simulink model "W01_Base_Map_cs"  (R2019a)
settings: Solver=FixedStepDiscrete  StartTime=0.0  StopTime=inf  FixedStep=1/20  RelTol=1e-3
PreLoadFcn:
  | mbxruntime.callbacks.PreLoadFcn(bdroot);
  | check_NUTS_defined
  | model_closed = 0;
  | assignin('base',['model_closed_' bdroot],false);
PostLoadFcn:
  | mbxruntime.callbacks.PostLoadFcn(bdroot);
InitFcn:
  | mbxruntime.callbacks.InitFcn(bdroot);
StartFcn:
  | mbxruntime.callbacks.StartFcn(bdroot);
StopFcn:
  | mbxruntime.callbacks.StopFcn(bdroot);;
  | 
model workspace: external: MAT-File .\W01_Base_Map_cs_hws.mat (data not in the file)
undefined symbols (not defined in the file or in its folder): DiscIntNeverNeededParam, Header, mbxruntime, Orientation, Poses, Poses_SL_Info, Position, tabledata, W01_Base_Map_cs_328ec7e3a8cd5b54, W01_Base_Map_cs_514c2dea2cdbe680, W01_Base_Map_cs_51d6e6e467bedba1, W01_Base_Map_cs_563ebd29d1fd6c09, W01_Base_Map_cs_57ea59d0358dab77, W01_Base_Map_cs_9538d35a279fbe4e, W01_Base_Map_cs_9f504bb84aebc2fd, W01_Base_Map_cs_a242ed7539861165, W01_Base_Map_cs_Audi_A8_Sedan_1_Path_pathUniqueID, W01_Base_Map_cs_b5931a786e299506, W01_Base_Map_cs_b7f45a070fa6e639, W01_Base_Map_cs_c02beb48492dde12, W01_Base_Map_cs_cf83ac8e8b053cbf, W01_Base_Map_cs_Child_RegularAni_1_Path_pathUniqueID, W01_Base_Map_cs_Child_RegularAni_2_Path_pathUniqueID, W01_Base_Map_cs_Citroen_C3_Hatchback_1_Path_pathUniqueID, W01_Base_Map_cs_d4423fcf1c0d6fc4, W01_Base_Map_cs_Female_RegularAni_1_Path_pathUniqueID, W01_Base_Map_cs_Male_RegularAni_1_Path_pathUniqueID, W01_Base_Map_cs_Male_RegularAni_2_Path_pathUniqueID
libraries: simulink_extras x30, adeye_lib x16, simulink x10, robotlib x4, sharedtransform x2, PreScanSimulinkLibrary x2, PreScanUsefulBlocks x1
(part 7 of 8)

== system W01_Base_Map_cs/TrafficLightRoadSideNL_1/Green_Mux ==
  MSCD [Cd] : Inport
  Position (xyz) [m] : Inport  Port=2
  Orientation (RPY) [deg] : Inport  Port=3
  Color [-] : Inport  Port=4
  TextureResourceID [-] : Inport  Port=5
  Bus Creator : BusCreator  Inputs='Intensity','Position','Orientation','Color','TextureResourceID'  OutDataTypeStr=Bus: PRESCAN_VISULIGHTACTUATOR_DATA  NonVirtualBus=on
  Bus Creator1 : BusCreator  Inputs=3  OutDataTypeStr=Bus: PRESCAN_RGB_DATA  NonVirtualBus=on
  Bus Creator2 : BusCreator  Inputs=3  OutDataTypeStr=Bus: PRESCAN_RPY_DATA  NonVirtualBus=on
  Bus Creator3 : BusCreator  Inputs=3  OutDataTypeStr=Bus: PRESCAN_XYZ_DATA  NonVirtualBus=on
  Data Type Conversion : DataTypeConversion  OutDataTypeStr=int32  RndMeth=Nearest
  Degrees to Radians : simulink_extras/Transformations/Degrees to Radians
  Demux : Demux  Outputs=3
  Demux1 : Demux  Outputs=3
  Demux2 : Demux  Outputs=3
  Lights : Outport
  wires:
  TextureResourceID [-]/1 -> Data Type Conversion/1  "TextureResourceID"
  MSCD [Cd]/1 -> Bus Creator/1  "Intensity"
  Bus Creator/1 -> Lights/1
  Demux/1 -> Bus Creator1/1  "R"
  Demux/2 -> Bus Creator1/2  "G"
  Demux/3 -> Bus Creator1/3  "B"
  Color [-]/1 -> Demux/1  "Color"
  Bus Creator1/1 -> Bus Creator/4  "Color"
  Demux1/1 -> Bus Creator2/1  "Roll"
  Demux1/2 -> Bus Creator2/2  "Pitch"
  Demux1/3 -> Bus Creator2/3  "Yaw"
  Orientation (RPY) [deg]/1 -> Degrees to Radians/1  "Orientation"
  Bus Creator2/1 -> Bus Creator/3  "Orientation"
  Demux2/1 -> Bus Creator3/1  "X"
  Demux2/2 -> Bus Creator3/2  "Y"
  Demux2/3 -> Bus Creator3/3  "Z"
  Position (xyz) [m]/1 -> Demux2/1  "Position"
  Bus Creator3/1 -> Bus Creator/2  "Position"
  Data Type Conversion/1 -> Bus Creator/5  "TextureResourceID"
  Degrees to Radians/1 -> Demux1/1

== system W01_Base_Map_cs/TrafficLightRoadSideNL_1/Orange_Mux ==
  MSCD [Cd] : Inport
  Position (xyz) [m] : Inport  Port=2
  Orientation (RPY) [deg] : Inport  Port=3
  Color [-] : Inport  Port=4
  TextureResourceID [-] : Inport  Port=5
  Bus Creator : BusCreator  Inputs='Intensity','Position','Orientation','Color','TextureResourceID'  OutDataTypeStr=Bus: PRESCAN_VISULIGHTACTUATOR_DATA  NonVirtualBus=on
  Bus Creator1 : BusCreator  Inputs=3  OutDataTypeStr=Bus: PRESCAN_RGB_DATA  NonVirtualBus=on
  Bus Creator2 : BusCreator  Inputs=3  OutDataTypeStr=Bus: PRESCAN_RPY_DATA  NonVirtualBus=on
  Bus Creator3 : BusCreator  Inputs=3  OutDataTypeStr=Bus: PRESCAN_XYZ_DATA  NonVirtualBus=on
  Data Type Conversion : DataTypeConversion  OutDataTypeStr=int32  RndMeth=Nearest
  Degrees to Radians : simulink_extras/Transformations/Degrees to Radians
  Demux : Demux  Outputs=3
  Demux1 : Demux  Outputs=3
  Demux2 : Demux  Outputs=3
  Lights : Outport
  wires:
  TextureResourceID [-]/1 -> Data Type Conversion/1  "TextureResourceID"
  MSCD [Cd]/1 -> Bus Creator/1  "Intensity"
  Bus Creator/1 -> Lights/1
  Demux/1 -> Bus Creator1/1  "R"
  Demux/2 -> Bus Creator1/2  "G"
  Demux/3 -> Bus Creator1/3  "B"
  Color [-]/1 -> Demux/1  "Color"
  Bus Creator1/1 -> Bus Creator/4  "Color"
  Demux1/1 -> Bus Creator2/1  "Roll"
  Demux1/2 -> Bus Creator2/2  "Pitch"
  Demux1/3 -> Bus Creator2/3  "Yaw"
  Orientation (RPY) [deg]/1 -> Degrees to Radians/1  "Orientation"
  Bus Creator2/1 -> Bus Creator/3  "Orientation"
  Demux2/1 -> Bus Creator3/1  "X"
  Demux2/2 -> Bus Creator3/2  "Y"
  Demux2/3 -> Bus Creator3/3  "Z"
  Position (xyz) [m]/1 -> Demux2/1  "Position"
  Bus Creator3/1 -> Bus Creator/2  "Position"
  Data Type Conversion/1 -> Bus Creator/5  "TextureResourceID"
  Degrees to Radians/1 -> Demux1/1

== system W01_Base_Map_cs/TrafficLightRoadSideNL_1/Red_Mux ==
  MSCD [Cd] : Inport
  Position (xyz) [m] : Inport  Port=2
  Orientation (RPY) [deg] : Inport  Port=3
  Color [-] : Inport  Port=4
  TextureResourceID [-] : Inport  Port=5
  Bus Creator : BusCreator  Inputs='Intensity','Position','Orientation','Color','TextureResourceID'  OutDataTypeStr=Bus: PRESCAN_VISULIGHTACTUATOR_DATA  NonVirtualBus=on
  Bus Creator1 : BusCreator  Inputs=3  OutDataTypeStr=Bus: PRESCAN_RGB_DATA  NonVirtualBus=on
  Bus Creator2 : BusCreator  Inputs=3  OutDataTypeStr=Bus: PRESCAN_RPY_DATA  NonVirtualBus=on
  Bus Creator3 : BusCreator  Inputs=3  OutDataTypeStr=Bus: PRESCAN_XYZ_DATA  NonVirtualBus=on
  Data Type Conversion : DataTypeConversion  OutDataTypeStr=int32  RndMeth=Nearest
  Degrees to Radians : simulink_extras/Transformations/Degrees to Radians
  Demux : Demux  Outputs=3
  Demux1 : Demux  Outputs=3
  Demux2 : Demux  Outputs=3
  Lights : Outport
  wires:
  TextureResourceID [-]/1 -> Data Type Conversion/1  "TextureResourceID"
  MSCD [Cd]/1 -> Bus Creator/1  "Intensity"
  Bus Creator/1 -> Lights/1
  Demux/1 -> Bus Creator1/1  "R"
  Demux/2 -> Bus Creator1/2  "G"
  Demux/3 -> Bus Creator1/3  "B"
  Color [-]/1 -> Demux/1  "Color"
  Bus Creator1/1 -> Bus Creator/4  "Color"
  Demux1/1 -> Bus Creator2/1  "Roll"
  Demux1/2 -> Bus Creator2/2  "Pitch"
  Demux1/3 -> Bus Creator2/3  "Yaw"
  Orientation (RPY) [deg]/1 -> Degrees to Radians/1  "Orientation"
  Bus Creator2/1 -> Bus Creator/3  "Orientation"
  Demux2/1 -> Bus Creator3/1  "X"
  Demux2/2 -> Bus Creator3/2  "Y"
  Demux2/3 -> Bus Creator3/3  "Z"
  Position (xyz) [m]/1 -> Demux2/1  "Position"
  Bus Creator3/1 -> Bus Creator/2  "Position"
  Data Type Conversion/1 -> Bus Creator/5  "TextureResourceID"
  Degrees to Radians/1 -> Demux1/1

== system W01_Base_Map_cs/TrafficLightRoadSideNL_2/Green_Mux ==
  MSCD [Cd] : Inport
  Position (xyz) [m] : Inport  Port=2
  Orientation (RPY) [deg] : Inport  Port=3
  Color [-] : Inport  Port=4
  TextureResourceID [-] : Inport  Port=5
  Bus Creator : BusCreator  Inputs='Intensity','Position','Orientation','Color','TextureResourceID'  OutDataTypeStr=Bus: PRESCAN_VISULIGHTACTUATOR_DATA  NonVirtualBus=on
  Bus Creator1 : BusCreator  Inputs=3  OutDataTypeStr=Bus: PRESCAN_RGB_DATA  NonVirtualBus=on
  Bus Creator2 : BusCreator  Inputs=3  OutDataTypeStr=Bus: PRESCAN_RPY_DATA  NonVirtualBus=on
  Bus Creator3 : BusCreator  Inputs=3  OutDataTypeStr=Bus: PRESCAN_XYZ_DATA  NonVirtualBus=on
  Data Type Conversion : DataTypeConversion  OutDataTypeStr=int32  RndMeth=Nearest
  Degrees to Radians : simulink_extras/Transformations/Degrees to Radians
  Demux : Demux  Outputs=3
  Demux1 : Demux  Outputs=3
  Demux2 : Demux  Outputs=3
  Lights : Outport
  wires:
  TextureResourceID [-]/1 -> Data Type Conversion/1  "TextureResourceID"
  MSCD [Cd]/1 -> Bus Creator/1  "Intensity"
  Bus Creator/1 -> Lights/1
  Demux/1 -> Bus Creator1/1  "R"
  Demux/2 -> Bus Creator1/2  "G"
  Demux/3 -> Bus Creator1/3  "B"
  Color [-]/1 -> Demux/1  "Color"
  Bus Creator1/1 -> Bus Creator/4  "Color"
  Demux1/1 -> Bus Creator2/1  "Roll"
  Demux1/2 -> Bus Creator2/2  "Pitch"
  Demux1/3 -> Bus Creator2/3  "Yaw"
  Orientation (RPY) [deg]/1 -> Degrees to Radians/1  "Orientation"
  Bus Creator2/1 -> Bus Creator/3  "Orientation"
  Demux2/1 -> Bus Creator3/1  "X"
  Demux2/2 -> Bus Creator3/2  "Y"
  Demux2/3 -> Bus Creator3/3  "Z"
  Position (xyz) [m]/1 -> Demux2/1  "Position"
  Bus Creator3/1 -> Bus Creator/2  "Position"
  Data Type Conversion/1 -> Bus Creator/5  "TextureResourceID"
  Degrees to Radians/1 -> Demux1/1

== system W01_Base_Map_cs/TrafficLightRoadSideNL_2/Orange_Mux ==
  MSCD [Cd] : Inport
  Position (xyz) [m] : Inport  Port=2
  Orientation (RPY) [deg] : Inport  Port=3
  Color [-] : Inport  Port=4
  TextureResourceID [-] : Inport  Port=5
  Bus Creator : BusCreator  Inputs='Intensity','Position','Orientation','Color','TextureResourceID'  OutDataTypeStr=Bus: PRESCAN_VISULIGHTACTUATOR_DATA  NonVirtualBus=on
  Bus Creator1 : BusCreator  Inputs=3  OutDataTypeStr=Bus: PRESCAN_RGB_DATA  NonVirtualBus=on
  Bus Creator2 : BusCreator  Inputs=3  OutDataTypeStr=Bus: PRESCAN_RPY_DATA  NonVirtualBus=on
  Bus Creator3 : BusCreator  Inputs=3  OutDataTypeStr=Bus: PRESCAN_XYZ_DATA  NonVirtualBus=on
  Data Type Conversion : DataTypeConversion  OutDataTypeStr=int32  RndMeth=Nearest
  Degrees to Radians : simulink_extras/Transformations/Degrees to Radians
  Demux : Demux  Outputs=3
  Demux1 : Demux  Outputs=3
  Demux2 : Demux  Outputs=3
  Lights : Outport
  wires:
  TextureResourceID [-]/1 -> Data Type Conversion/1  "TextureResourceID"
  MSCD [Cd]/1 -> Bus Creator/1  "Intensity"
  Bus Creator/1 -> Lights/1
  Demux/1 -> Bus Creator1/1  "R"
  Demux/2 -> Bus Creator1/2  "G"
  Demux/3 -> Bus Creator1/3  "B"
  Color [-]/1 -> Demux/1  "Color"
  Bus Creator1/1 -> Bus Creator/4  "Color"
  Demux1/1 -> Bus Creator2/1  "Roll"
  Demux1/2 -> Bus Creator2/2  "Pitch"
  Demux1/3 -> Bus Creator2/3  "Yaw"
  Orientation (RPY) [deg]/1 -> Degrees to Radians/1  "Orientation"
  Bus Creator2/1 -> Bus Creator/3  "Orientation"
  Demux2/1 -> Bus Creator3/1  "X"
  Demux2/2 -> Bus Creator3/2  "Y"
  Demux2/3 -> Bus Creator3/3  "Z"
  Position (xyz) [m]/1 -> Demux2/1  "Position"
  Bus Creator3/1 -> Bus Creator/2  "Position"
  Data Type Conversion/1 -> Bus Creator/5  "TextureResourceID"
  Degrees to Radians/1 -> Demux1/1

== system W01_Base_Map_cs/TrafficLightRoadSideNL_2/Red_Mux ==
  MSCD [Cd] : Inport
  Position (xyz) [m] : Inport  Port=2
  Orientation (RPY) [deg] : Inport  Port=3
  Color [-] : Inport  Port=4
  TextureResourceID [-] : Inport  Port=5
  Bus Creator : BusCreator  Inputs='Intensity','Position','Orientation','Color','TextureResourceID'  OutDataTypeStr=Bus: PRESCAN_VISULIGHTACTUATOR_DATA  NonVirtualBus=on
  Bus Creator1 : BusCreator  Inputs=3  OutDataTypeStr=Bus: PRESCAN_RGB_DATA  NonVirtualBus=on
  Bus Creator2 : BusCreator  Inputs=3  OutDataTypeStr=Bus: PRESCAN_RPY_DATA  NonVirtualBus=on
  Bus Creator3 : BusCreator  Inputs=3  OutDataTypeStr=Bus: PRESCAN_XYZ_DATA  NonVirtualBus=on
  Data Type Conversion : DataTypeConversion  OutDataTypeStr=int32  RndMeth=Nearest
  Degrees to Radians : simulink_extras/Transformations/Degrees to Radians
  Demux : Demux  Outputs=3
  Demux1 : Demux  Outputs=3
  Demux2 : Demux  Outputs=3
  Lights : Outport
  wires:
  TextureResourceID [-]/1 -> Data Type Conversion/1  "TextureResourceID"
  MSCD [Cd]/1 -> Bus Creator/1  "Intensity"
  Bus Creator/1 -> Lights/1
  Demux/1 -> Bus Creator1/1  "R"
  Demux/2 -> Bus Creator1/2  "G"
  Demux/3 -> Bus Creator1/3  "B"
  Color [-]/1 -> Demux/1  "Color"
  Bus Creator1/1 -> Bus Creator/4  "Color"
  Demux1/1 -> Bus Creator2/1  "Roll"
  Demux1/2 -> Bus Creator2/2  "Pitch"
  Demux1/3 -> Bus Creator2/3  "Yaw"
  Orientation (RPY) [deg]/1 -> Degrees to Radians/1  "Orientation"
  Bus Creator2/1 -> Bus Creator/3  "Orientation"
  Demux2/1 -> Bus Creator3/1  "X"
  Demux2/2 -> Bus Creator3/2  "Y"
  Demux2/3 -> Bus Creator3/3  "Z"
  Position (xyz) [m]/1 -> Demux2/1  "Position"
  Bus Creator3/1 -> Bus Creator/2  "Position"
  Data Type Conversion/1 -> Bus Creator/5  "TextureResourceID"
  Degrees to Radians/1 -> Demux1/1

== system W01_Base_Map_cs/TrafficLightRoadSideNL_3/Green_Mux ==
  MSCD [Cd] : Inport
  Position (xyz) [m] : Inport  Port=2
  Orientation (RPY) [deg] : Inport  Port=3
  Color [-] : Inport  Port=4
  TextureResourceID [-] : Inport  Port=5
  Bus Creator : BusCreator  Inputs='Intensity','Position','Orientation','Color','TextureResourceID'  OutDataTypeStr=Bus: PRESCAN_VISULIGHTACTUATOR_DATA  NonVirtualBus=on
  Bus Creator1 : BusCreator  Inputs=3  OutDataTypeStr=Bus: PRESCAN_RGB_DATA  NonVirtualBus=on
  Bus Creator2 : BusCreator  Inputs=3  OutDataTypeStr=Bus: PRESCAN_RPY_DATA  NonVirtualBus=on
  Bus Creator3 : BusCreator  Inputs=3  OutDataTypeStr=Bus: PRESCAN_XYZ_DATA  NonVirtualBus=on
  Data Type Conversion : DataTypeConversion  OutDataTypeStr=int32  RndMeth=Nearest
  Degrees to Radians : simulink_extras/Transformations/Degrees to Radians
  Demux : Demux  Outputs=3
  Demux1 : Demux  Outputs=3
  Demux2 : Demux  Outputs=3
  Lights : Outport
  wires:
  TextureResourceID [-]/1 -> Data Type Conversion/1  "TextureResourceID"
  MSCD [Cd]/1 -> Bus Creator/1  "Intensity"
  Bus Creator/1 -> Lights/1
  Demux/1 -> Bus Creator1/1  "R"
  Demux/2 -> Bus Creator1/2  "G"
  Demux/3 -> Bus Creator1/3  "B"
  Color [-]/1 -> Demux/1  "Color"
  Bus Creator1/1 -> Bus Creator/4  "Color"
  Demux1/1 -> Bus Creator2/1  "Roll"
  Demux1/2 -> Bus Creator2/2  "Pitch"
  Demux1/3 -> Bus Creator2/3  "Yaw"
  Orientation (RPY) [deg]/1 -> Degrees to Radians/1  "Orientation"
  Bus Creator2/1 -> Bus Creator/3  "Orientation"
  Demux2/1 -> Bus Creator3/1  "X"
  Demux2/2 -> Bus Creator3/2  "Y"
  Demux2/3 -> Bus Creator3/3  "Z"
  Position (xyz) [m]/1 -> Demux2/1  "Position"
  Bus Creator3/1 -> Bus Creator/2  "Position"
  Data Type Conversion/1 -> Bus Creator/5  "TextureResourceID"
  Degrees to Radians/1 -> Demux1/1

== system W01_Base_Map_cs/TrafficLightRoadSideNL_3/Orange_Mux ==
  MSCD [Cd] : Inport
  Position (xyz) [m] : Inport  Port=2
  Orientation (RPY) [deg] : Inport  Port=3
  Color [-] : Inport  Port=4
  TextureResourceID [-] : Inport  Port=5
  Bus Creator : BusCreator  Inputs='Intensity','Position','Orientation','Color','TextureResourceID'  OutDataTypeStr=Bus: PRESCAN_VISULIGHTACTUATOR_DATA  NonVirtualBus=on
  Bus Creator1 : BusCreator  Inputs=3  OutDataTypeStr=Bus: PRESCAN_RGB_DATA  NonVirtualBus=on
  Bus Creator2 : BusCreator  Inputs=3  OutDataTypeStr=Bus: PRESCAN_RPY_DATA  NonVirtualBus=on
  Bus Creator3 : BusCreator  Inputs=3  OutDataTypeStr=Bus: PRESCAN_XYZ_DATA  NonVirtualBus=on
  Data Type Conversion : DataTypeConversion  OutDataTypeStr=int32  RndMeth=Nearest
  Degrees to Radians : simulink_extras/Transformations/Degrees to Radians
  Demux : Demux  Outputs=3
  Demux1 : Demux  Outputs=3
  Demux2 : Demux  Outputs=3
  Lights : Outport
  wires:
  TextureResourceID [-]/1 -> Data Type Conversion/1  "TextureResourceID"
  MSCD [Cd]/1 -> Bus Creator/1  "Intensity"
  Bus Creator/1 -> Lights/1
  Demux/1 -> Bus Creator1/1  "R"
  Demux/2 -> Bus Creator1/2  "G"
  Demux/3 -> Bus Creator1/3  "B"
  Color [-]/1 -> Demux/1  "Color"
  Bus Creator1/1 -> Bus Creator/4  "Color"
  Demux1/1 -> Bus Creator2/1  "Roll"
  Demux1/2 -> Bus Creator2/2  "Pitch"
  Demux1/3 -> Bus Creator2/3  "Yaw"
  Orientation (RPY) [deg]/1 -> Degrees to Radians/1  "Orientation"
  Bus Creator2/1 -> Bus Creator/3  "Orientation"
  Demux2/1 -> Bus Creator3/1  "X"
  Demux2/2 -> Bus Creator3/2  "Y"
  Demux2/3 -> Bus Creator3/3  "Z"
  Position (xyz) [m]/1 -> Demux2/1  "Position"
  Bus Creator3/1 -> Bus Creator/2  "Position"
  Data Type Conversion/1 -> Bus Creator/5  "TextureResourceID"
  Degrees to Radians/1 -> Demux1/1

== system W01_Base_Map_cs/TrafficLightRoadSideNL_3/Red_Mux ==
  MSCD [Cd] : Inport
  Position (xyz) [m] : Inport  Port=2
  Orientation (RPY) [deg] : Inport  Port=3
  Color [-] : Inport  Port=4
  TextureResourceID [-] : Inport  Port=5
  Bus Creator : BusCreator  Inputs='Intensity','Position','Orientation','Color','TextureResourceID'  OutDataTypeStr=Bus: PRESCAN_VISULIGHTACTUATOR_DATA  NonVirtualBus=on
  Bus Creator1 : BusCreator  Inputs=3  OutDataTypeStr=Bus: PRESCAN_RGB_DATA  NonVirtualBus=on
  Bus Creator2 : BusCreator  Inputs=3  OutDataTypeStr=Bus: PRESCAN_RPY_DATA  NonVirtualBus=on
  Bus Creator3 : BusCreator  Inputs=3  OutDataTypeStr=Bus: PRESCAN_XYZ_DATA  NonVirtualBus=on
  Data Type Conversion : DataTypeConversion  OutDataTypeStr=int32  RndMeth=Nearest
  Degrees to Radians : simulink_extras/Transformations/Degrees to Radians
  Demux : Demux  Outputs=3
  Demux1 : Demux  Outputs=3
  Demux2 : Demux  Outputs=3
  Lights : Outport
  wires:
  TextureResourceID [-]/1 -> Data Type Conversion/1  "TextureResourceID"
  MSCD [Cd]/1 -> Bus Creator/1  "Intensity"
  Bus Creator/1 -> Lights/1
  Demux/1 -> Bus Creator1/1  "R"
  Demux/2 -> Bus Creator1/2  "G"
  Demux/3 -> Bus Creator1/3  "B"
  Color [-]/1 -> Demux/1  "Color"
  Bus Creator1/1 -> Bus Creator/4  "Color"
  Demux1/1 -> Bus Creator2/1  "Roll"
  Demux1/2 -> Bus Creator2/2  "Pitch"
  Demux1/3 -> Bus Creator2/3  "Yaw"
  Orientation (RPY) [deg]/1 -> Degrees to Radians/1  "Orientation"
  Bus Creator2/1 -> Bus Creator/3  "Orientation"
  Demux2/1 -> Bus Creator3/1  "X"
  Demux2/2 -> Bus Creator3/2  "Y"
  Demux2/3 -> Bus Creator3/3  "Z"
  Position (xyz) [m]/1 -> Demux2/1  "Position"
  Bus Creator3/1 -> Bus Creator/2  "Position"
  Data Type Conversion/1 -> Bus Creator/5  "TextureResourceID"
  Degrees to Radians/1 -> Demux1/1

== system W01_Base_Map_cs/TrafficLightRoadSideNL_4/Green_Mux ==
  MSCD [Cd] : Inport
  Position (xyz) [m] : Inport  Port=2
  Orientation (RPY) [deg] : Inport  Port=3
  Color [-] : Inport  Port=4
  TextureResourceID [-] : Inport  Port=5
  Bus Creator : BusCreator  Inputs='Intensity','Position','Orientation','Color','TextureResourceID'  OutDataTypeStr=Bus: PRESCAN_VISULIGHTACTUATOR_DATA  NonVirtualBus=on
  Bus Creator1 : BusCreator  Inputs=3  OutDataTypeStr=Bus: PRESCAN_RGB_DATA  NonVirtualBus=on
  Bus Creator2 : BusCreator  Inputs=3  OutDataTypeStr=Bus: PRESCAN_RPY_DATA  NonVirtualBus=on
  Bus Creator3 : BusCreator  Inputs=3  OutDataTypeStr=Bus: PRESCAN_XYZ_DATA  NonVirtualBus=on
  Data Type Conversion : DataTypeConversion  OutDataTypeStr=int32  RndMeth=Nearest
  Degrees to Radians : simulink_extras/Transformations/Degrees to Radians
  Demux : Demux  Outputs=3
  Demux1 : Demux  Outputs=3
  Demux2 : Demux  Outputs=3
  Lights : Outport
  wires:
  TextureResourceID [-]/1 -> Data Type Conversion/1  "TextureResourceID"
  MSCD [Cd]/1 -> Bus Creator/1  "Intensity"
  Bus Creator/1 -> Lights/1
  Demux/1 -> Bus Creator1/1  "R"
  Demux/2 -> Bus Creator1/2  "G"
  Demux/3 -> Bus Creator1/3  "B"
  Color [-]/1 -> Demux/1  "Color"
  Bus Creator1/1 -> Bus Creator/4  "Color"
  Demux1/1 -> Bus Creator2/1  "Roll"
  Demux1/2 -> Bus Creator2/2  "Pitch"
  Demux1/3 -> Bus Creator2/3  "Yaw"
  Orientation (RPY) [deg]/1 -> Degrees to Radians/1  "Orientation"
  Bus Creator2/1 -> Bus Creator/3  "Orientation"
  Demux2/1 -> Bus Creator3/1  "X"
  Demux2/2 -> Bus Creator3/2  "Y"
  Demux2/3 -> Bus Creator3/3  "Z"
  Position (xyz) [m]/1 -> Demux2/1  "Position"
  Bus Creator3/1 -> Bus Creator/2  "Position"
  Data Type Conversion/1 -> Bus Creator/5  "TextureResourceID"
  Degrees to Radians/1 -> Demux1/1

== system W01_Base_Map_cs/TrafficLightRoadSideNL_4/Orange_Mux ==
  MSCD [Cd] : Inport
  Position (xyz) [m] : Inport  Port=2
  Orientation (RPY) [deg] : Inport  Port=3
  Color [-] : Inport  Port=4
  TextureResourceID [-] : Inport  Port=5
  Bus Creator : BusCreator  Inputs='Intensity','Position','Orientation','Color','TextureResourceID'  OutDataTypeStr=Bus: PRESCAN_VISULIGHTACTUATOR_DATA  NonVirtualBus=on
  Bus Creator1 : BusCreator  Inputs=3  OutDataTypeStr=Bus: PRESCAN_RGB_DATA  NonVirtualBus=on
  Bus Creator2 : BusCreator  Inputs=3  OutDataTypeStr=Bus: PRESCAN_RPY_DATA  NonVirtualBus=on
  Bus Creator3 : BusCreator  Inputs=3  OutDataTypeStr=Bus: PRESCAN_XYZ_DATA  NonVirtualBus=on
  Data Type Conversion : DataTypeConversion  OutDataTypeStr=int32  RndMeth=Nearest
  Degrees to Radians : simulink_extras/Transformations/Degrees to Radians
  Demux : Demux  Outputs=3
  Demux1 : Demux  Outputs=3
  Demux2 : Demux  Outputs=3
  Lights : Outport
  wires:
  TextureResourceID [-]/1 -> Data Type Conversion/1  "TextureResourceID"
  MSCD [Cd]/1 -> Bus Creator/1  "Intensity"
  Bus Creator/1 -> Lights/1
  Demux/1 -> Bus Creator1/1  "R"
  Demux/2 -> Bus Creator1/2  "G"
  Demux/3 -> Bus Creator1/3  "B"
  Color [-]/1 -> Demux/1  "Color"
  Bus Creator1/1 -> Bus Creator/4  "Color"
  Demux1/1 -> Bus Creator2/1  "Roll"
  Demux1/2 -> Bus Creator2/2  "Pitch"
  Demux1/3 -> Bus Creator2/3  "Yaw"
  Orientation (RPY) [deg]/1 -> Degrees to Radians/1  "Orientation"
  Bus Creator2/1 -> Bus Creator/3  "Orientation"
  Demux2/1 -> Bus Creator3/1  "X"
  Demux2/2 -> Bus Creator3/2  "Y"
  Demux2/3 -> Bus Creator3/3  "Z"
  Position (xyz) [m]/1 -> Demux2/1  "Position"
  Bus Creator3/1 -> Bus Creator/2  "Position"
  Data Type Conversion/1 -> Bus Creator/5  "TextureResourceID"
  Degrees to Radians/1 -> Demux1/1

== system W01_Base_Map_cs/TrafficLightRoadSideNL_4/Red_Mux ==
  MSCD [Cd] : Inport
  Position (xyz) [m] : Inport  Port=2
  Orientation (RPY) [deg] : Inport  Port=3
  Color [-] : Inport  Port=4
  TextureResourceID [-] : Inport  Port=5
  Bus Creator : BusCreator  Inputs='Intensity','Position','Orientation','Color','TextureResourceID'  OutDataTypeStr=Bus: PRESCAN_VISULIGHTACTUATOR_DATA  NonVirtualBus=on
  Bus Creator1 : BusCreator  Inputs=3  OutDataTypeStr=Bus: PRESCAN_RGB_DATA  NonVirtualBus=on
  Bus Creator2 : BusCreator  Inputs=3  OutDataTypeStr=Bus: PRESCAN_RPY_DATA  NonVirtualBus=on
  Bus Creator3 : BusCreator  Inputs=3  OutDataTypeStr=Bus: PRESCAN_XYZ_DATA  NonVirtualBus=on
  Data Type Conversion : DataTypeConversion  OutDataTypeStr=int32  RndMeth=Nearest
  Degrees to Radians : simulink_extras/Transformations/Degrees to Radians
  Demux : Demux  Outputs=3
  Demux1 : Demux  Outputs=3
  Demux2 : Demux  Outputs=3
  Lights : Outport
  wires:
  TextureResourceID [-]/1 -> Data Type Conversion/1  "TextureResourceID"
  MSCD [Cd]/1 -> Bus Creator/1  "Intensity"
  Bus Creator/1 -> Lights/1
  Demux/1 -> Bus Creator1/1  "R"
  Demux/2 -> Bus Creator1/2  "G"
  Demux/3 -> Bus Creator1/3  "B"
  Color [-]/1 -> Demux/1  "Color"
  Bus Creator1/1 -> Bus Creator/4  "Color"
  Demux1/1 -> Bus Creator2/1  "Roll"
  Demux1/2 -> Bus Creator2/2  "Pitch"
  Demux1/3 -> Bus Creator2/3  "Yaw"
  Orientation (RPY) [deg]/1 -> Degrees to Radians/1  "Orientation"
  Bus Creator2/1 -> Bus Creator/3  "Orientation"
  Demux2/1 -> Bus Creator3/1  "X"
  Demux2/2 -> Bus Creator3/2  "Y"
  Demux2/3 -> Bus Creator3/3  "Z"
  Position (xyz) [m]/1 -> Demux2/1  "Position"
  Bus Creator3/1 -> Bus Creator/2  "Position"
  Data Type Conversion/1 -> Bus Creator/5  "TextureResourceID"
  Degrees to Radians/1 -> Demux1/1

== system W01_Base_Map_cs/TrafficLightRoadSideNL_5/Green_Mux ==
  MSCD [Cd] : Inport
  Position (xyz) [m] : Inport  Port=2
  Orientation (RPY) [deg] : Inport  Port=3
  Color [-] : Inport  Port=4
  TextureResourceID [-] : Inport  Port=5
  Bus Creator : BusCreator  Inputs='Intensity','Position','Orientation','Color','TextureResourceID'  OutDataTypeStr=Bus: PRESCAN_VISULIGHTACTUATOR_DATA  NonVirtualBus=on
  Bus Creator1 : BusCreator  Inputs=3  OutDataTypeStr=Bus: PRESCAN_RGB_DATA  NonVirtualBus=on
  Bus Creator2 : BusCreator  Inputs=3  OutDataTypeStr=Bus: PRESCAN_RPY_DATA  NonVirtualBus=on
  Bus Creator3 : BusCreator  Inputs=3  OutDataTypeStr=Bus: PRESCAN_XYZ_DATA  NonVirtualBus=on
  Data Type Conversion : DataTypeConversion  OutDataTypeStr=int32  RndMeth=Nearest
  Degrees to Radians : simulink_extras/Transformations/Degrees to Radians
  Demux : Demux  Outputs=3
  Demux1 : Demux  Outputs=3
  Demux2 : Demux  Outputs=3
  Lights : Outport
  wires:
  TextureResourceID [-]/1 -> Data Type Conversion/1  "TextureResourceID"
  MSCD [Cd]/1 -> Bus Creator/1  "Intensity"
  Bus Creator/1 -> Lights/1
  Demux/1 -> Bus Creator1/1  "R"
  Demux/2 -> Bus Creator1/2  "G"
  Demux/3 -> Bus Creator1/3  "B"
  Color [-]/1 -> Demux/1  "Color"
  Bus Creator1/1 -> Bus Creator/4  "Color"
  Demux1/1 -> Bus Creator2/1  "Roll"
  Demux1/2 -> Bus Creator2/2  "Pitch"
  Demux1/3 -> Bus Creator2/3  "Yaw"
  Orientation (RPY) [deg]/1 -> Degrees to Radians/1  "Orientation"
  Bus Creator2/1 -> Bus Creator/3  "Orientation"
  Demux2/1 -> Bus Creator3/1  "X"
  Demux2/2 -> Bus Creator3/2  "Y"
  Demux2/3 -> Bus Creator3/3  "Z"
  Position (xyz) [m]/1 -> Demux2/1  "Position"
  Bus Creator3/1 -> Bus Creator/2  "Position"
  Data Type Conversion/1 -> Bus Creator/5  "TextureResourceID"
  Degrees to Radians/1 -> Demux1/1

== system W01_Base_Map_cs/TrafficLightRoadSideNL_5/Orange_Mux ==
  MSCD [Cd] : Inport
  Position (xyz) [m] : Inport  Port=2
  Orientation (RPY) [deg] : Inport  Port=3
  Color [-] : Inport  Port=4
  TextureResourceID [-] : Inport  Port=5
  Bus Creator : BusCreator  Inputs='Intensity','Position','Orientation','Color','TextureResourceID'  OutDataTypeStr=Bus: PRESCAN_VISULIGHTACTUATOR_DATA  NonVirtualBus=on
  Bus Creator1 : BusCreator  Inputs=3  OutDataTypeStr=Bus: PRESCAN_RGB_DATA  NonVirtualBus=on
  Bus Creator2 : BusCreator  Inputs=3  OutDataTypeStr=Bus: PRESCAN_RPY_DATA  NonVirtualBus=on
  Bus Creator3 : BusCreator  Inputs=3  OutDataTypeStr=Bus: PRESCAN_XYZ_DATA  NonVirtualBus=on
  Data Type Conversion : DataTypeConversion  OutDataTypeStr=int32  RndMeth=Nearest
  Degrees to Radians : simulink_extras/Transformations/Degrees to Radians
  Demux : Demux  Outputs=3
  Demux1 : Demux  Outputs=3
  Demux2 : Demux  Outputs=3
  Lights : Outport
  wires:
  TextureResourceID [-]/1 -> Data Type Conversion/1  "TextureResourceID"
  MSCD [Cd]/1 -> Bus Creator/1  "Intensity"
  Bus Creator/1 -> Lights/1
  Demux/1 -> Bus Creator1/1  "R"
  Demux/2 -> Bus Creator1/2  "G"
  Demux/3 -> Bus Creator1/3  "B"
  Color [-]/1 -> Demux/1  "Color"
  Bus Creator1/1 -> Bus Creator/4  "Color"
  Demux1/1 -> Bus Creator2/1  "Roll"
  Demux1/2 -> Bus Creator2/2  "Pitch"
  Demux1/3 -> Bus Creator2/3  "Yaw"
  Orientation (RPY) [deg]/1 -> Degrees to Radians/1  "Orientation"
  Bus Creator2/1 -> Bus Creator/3  "Orientation"
  Demux2/1 -> Bus Creator3/1  "X"
  Demux2/2 -> Bus Creator3/2  "Y"
  Demux2/3 -> Bus Creator3/3  "Z"
  Position (xyz) [m]/1 -> Demux2/1  "Position"
  Bus Creator3/1 -> Bus Creator/2  "Position"
  Data Type Conversion/1 -> Bus Creator/5  "TextureResourceID"
  Degrees to Radians/1 -> Demux1/1

== system W01_Base_Map_cs/TrafficLightRoadSideNL_5/Red_Mux ==
  MSCD [Cd] : Inport
  Position (xyz) [m] : Inport  Port=2
  Orientation (RPY) [deg] : Inport  Port=3
  Color [-] : Inport  Port=4
  TextureResourceID [-] : Inport  Port=5
  Bus Creator : BusCreator  Inputs='Intensity','Position','Orientation','Color','TextureResourceID'  OutDataTypeStr=Bus: PRESCAN_VISULIGHTACTUATOR_DATA  NonVirtualBus=on
  Bus Creator1 : BusCreator  Inputs=3  OutDataTypeStr=Bus: PRESCAN_RGB_DATA  NonVirtualBus=on
  Bus Creator2 : BusCreator  Inputs=3  OutDataTypeStr=Bus: PRESCAN_RPY_DATA  NonVirtualBus=on
  Bus Creator3 : BusCreator  Inputs=3  OutDataTypeStr=Bus: PRESCAN_XYZ_DATA  NonVirtualBus=on
  Data Type Conversion : DataTypeConversion  OutDataTypeStr=int32  RndMeth=Nearest
  Degrees to Radians : simulink_extras/Transformations/Degrees to Radians
  Demux : Demux  Outputs=3
  Demux1 : Demux  Outputs=3
  Demux2 : Demux  Outputs=3
  Lights : Outport
  wires:
  TextureResourceID [-]/1 -> Data Type Conversion/1  "TextureResourceID"
  MSCD [Cd]/1 -> Bus Creator/1  "Intensity"
  Bus Creator/1 -> Lights/1
  Demux/1 -> Bus Creator1/1  "R"
  Demux/2 -> Bus Creator1/2  "G"
  Demux/3 -> Bus Creator1/3  "B"
  Color [-]/1 -> Demux/1  "Color"
  Bus Creator1/1 -> Bus Creator/4  "Color"
  Demux1/1 -> Bus Creator2/1  "Roll"
  Demux1/2 -> Bus Creator2/2  "Pitch"
  Demux1/3 -> Bus Creator2/3  "Yaw"
  Orientation (RPY) [deg]/1 -> Degrees to Radians/1  "Orientation"
  Bus Creator2/1 -> Bus Creator/3  "Orientation"
  Demux2/1 -> Bus Creator3/1  "X"
  Demux2/2 -> Bus Creator3/2  "Y"
  Demux2/3 -> Bus Creator3/3  "Z"
  Position (xyz) [m]/1 -> Demux2/1  "Position"
  Bus Creator3/1 -> Bus Creator/2  "Position"
  Data Type Conversion/1 -> Bus Creator/5  "TextureResourceID"
  Degrees to Radians/1 -> Demux1/1

== system W01_Base_Map_cs/TrafficLightRoadSideNL_6/Green_Mux ==
  MSCD [Cd] : Inport
  Position (xyz) [m] : Inport  Port=2
  Orientation (RPY) [deg] : Inport  Port=3
  Color [-] : Inport  Port=4
  TextureResourceID [-] : Inport  Port=5
  Bus Creator : BusCreator  Inputs='Intensity','Position','Orientation','Color','TextureResourceID'  OutDataTypeStr=Bus: PRESCAN_VISULIGHTACTUATOR_DATA  NonVirtualBus=on
  Bus Creator1 : BusCreator  Inputs=3  OutDataTypeStr=Bus: PRESCAN_RGB_DATA  NonVirtualBus=on
  Bus Creator2 : BusCreator  Inputs=3  OutDataTypeStr=Bus: PRESCAN_RPY_DATA  NonVirtualBus=on
  Bus Creator3 : BusCreator  Inputs=3  OutDataTypeStr=Bus: PRESCAN_XYZ_DATA  NonVirtualBus=on
  Data Type Conversion : DataTypeConversion  OutDataTypeStr=int32  RndMeth=Nearest
  Degrees to Radians : simulink_extras/Transformations/Degrees to Radians
  Demux : Demux  Outputs=3
  Demux1 : Demux  Outputs=3
  Demux2 : Demux  Outputs=3
  Lights : Outport
  wires:
  TextureResourceID [-]/1 -> Data Type Conversion/1  "TextureResourceID"
  MSCD [Cd]/1 -> Bus Creator/1  "Intensity"
  Bus Creator/1 -> Lights/1
  Demux/1 -> Bus Creator1/1  "R"
  Demux/2 -> Bus Creator1/2  "G"
  Demux/3 -> Bus Creator1/3  "B"
  Color [-]/1 -> Demux/1  "Color"
  Bus Creator1/1 -> Bus Creator/4  "Color"
  Demux1/1 -> Bus Creator2/1  "Roll"
  Demux1/2 -> Bus Creator2/2  "Pitch"
  Demux1/3 -> Bus Creator2/3  "Yaw"
  Orientation (RPY) [deg]/1 -> Degrees to Radians/1  "Orientation"
  Bus Creator2/1 -> Bus Creator/3  "Orientation"
  Demux2/1 -> Bus Creator3/1  "X"
  Demux2/2 -> Bus Creator3/2  "Y"
  Demux2/3 -> Bus Creator3/3  "Z"
  Position (xyz) [m]/1 -> Demux2/1  "Position"
  Bus Creator3/1 -> Bus Creator/2  "Position"
  Data Type Conversion/1 -> Bus Creator/5  "TextureResourceID"
  Degrees to Radians/1 -> Demux1/1

== system W01_Base_Map_cs/TrafficLightRoadSideNL_6/Orange_Mux ==
  MSCD [Cd] : Inport
  Position (xyz) [m] : Inport  Port=2
  Orientation (RPY) [deg] : Inport  Port=3
  Color [-] : Inport  Port=4
  TextureResourceID [-] : Inport  Port=5
  Bus Creator : BusCreator  Inputs='Intensity','Position','Orientation','Color','TextureResourceID'  OutDataTypeStr=Bus: PRESCAN_VISULIGHTACTUATOR_DATA  NonVirtualBus=on
  Bus Creator1 : BusCreator  Inputs=3  OutDataTypeStr=Bus: PRESCAN_RGB_DATA  NonVirtualBus=on
  Bus Creator2 : BusCreator  Inputs=3  OutDataTypeStr=Bus: PRESCAN_RPY_DATA  NonVirtualBus=on
  Bus Creator3 : BusCreator  Inputs=3  OutDataTypeStr=Bus: PRESCAN_XYZ_DATA  NonVirtualBus=on
  Data Type Conversion : DataTypeConversion  OutDataTypeStr=int32  RndMeth=Nearest
  Degrees to Radians : simulink_extras/Transformations/Degrees to Radians
  Demux : Demux  Outputs=3
  Demux1 : Demux  Outputs=3
  Demux2 : Demux  Outputs=3
  Lights : Outport
  wires:
  TextureResourceID [-]/1 -> Data Type Conversion/1  "TextureResourceID"
  MSCD [Cd]/1 -> Bus Creator/1  "Intensity"
  Bus Creator/1 -> Lights/1
  Demux/1 -> Bus Creator1/1  "R"
  Demux/2 -> Bus Creator1/2  "G"
  Demux/3 -> Bus Creator1/3  "B"
  Color [-]/1 -> Demux/1  "Color"
  Bus Creator1/1 -> Bus Creator/4  "Color"
  Demux1/1 -> Bus Creator2/1  "Roll"
  Demux1/2 -> Bus Creator2/2  "Pitch"
  Demux1/3 -> Bus Creator2/3  "Yaw"
  Orientation (RPY) [deg]/1 -> Degrees to Radians/1  "Orientation"
  Bus Creator2/1 -> Bus Creator/3  "Orientation"
  Demux2/1 -> Bus Creator3/1  "X"
  Demux2/2 -> Bus Creator3/2  "Y"
  Demux2/3 -> Bus Creator3/3  "Z"
  Position (xyz) [m]/1 -> Demux2/1  "Position"
  Bus Creator3/1 -> Bus Creator/2  "Position"
  Data Type Conversion/1 -> Bus Creator/5  "TextureResourceID"
  Degrees to Radians/1 -> Demux1/1

== system W01_Base_Map_cs/TrafficLightRoadSideNL_6/Red_Mux ==
  MSCD [Cd] : Inport
  Position (xyz) [m] : Inport  Port=2
  Orientation (RPY) [deg] : Inport  Port=3
  Color [-] : Inport  Port=4
  TextureResourceID [-] : Inport  Port=5
  Bus Creator : BusCreator  Inputs='Intensity','Position','Orientation','Color','TextureResourceID'  OutDataTypeStr=Bus: PRESCAN_VISULIGHTACTUATOR_DATA  NonVirtualBus=on
  Bus Creator1 : BusCreator  Inputs=3  OutDataTypeStr=Bus: PRESCAN_RGB_DATA  NonVirtualBus=on
  Bus Creator2 : BusCreator  Inputs=3  OutDataTypeStr=Bus: PRESCAN_RPY_DATA  NonVirtualBus=on
  Bus Creator3 : BusCreator  Inputs=3  OutDataTypeStr=Bus: PRESCAN_XYZ_DATA  NonVirtualBus=on
  Data Type Conversion : DataTypeConversion  OutDataTypeStr=int32  RndMeth=Nearest
  Degrees to Radians : simulink_extras/Transformations/Degrees to Radians
  Demux : Demux  Outputs=3
  Demux1 : Demux  Outputs=3
  Demux2 : Demux  Outputs=3
  Lights : Outport
  wires:
  TextureResourceID [-]/1 -> Data Type Conversion/1  "TextureResourceID"
  MSCD [Cd]/1 -> Bus Creator/1  "Intensity"
  Bus Creator/1 -> Lights/1
  Demux/1 -> Bus Creator1/1  "R"
  Demux/2 -> Bus Creator1/2  "G"
  Demux/3 -> Bus Creator1/3  "B"
  Color [-]/1 -> Demux/1  "Color"
  Bus Creator1/1 -> Bus Creator/4  "Color"
  Demux1/1 -> Bus Creator2/1  "Roll"
  Demux1/2 -> Bus Creator2/2  "Pitch"
  Demux1/3 -> Bus Creator2/3  "Yaw"
  Orientation (RPY) [deg]/1 -> Degrees to Radians/1  "Orientation"
  Bus Creator2/1 -> Bus Creator/3  "Orientation"
  Demux2/1 -> Bus Creator3/1  "X"
  Demux2/2 -> Bus Creator3/2  "Y"
  Demux2/3 -> Bus Creator3/3  "Z"
  Position (xyz) [m]/1 -> Demux2/1  "Position"
  Bus Creator3/1 -> Bus Creator/2  "Position"
  Data Type Conversion/1 -> Bus Creator/5  "TextureResourceID"
  Degrees to Radians/1 -> Demux1/1

== system W01_Base_Map_cs/TrafficLightRoadSideNL_7/Green_Mux ==
  MSCD [Cd] : Inport
  Position (xyz) [m] : Inport  Port=2
  Orientation (RPY) [deg] : Inport  Port=3
  Color [-] : Inport  Port=4
  TextureResourceID [-] : Inport  Port=5
  Bus Creator : BusCreator  Inputs='Intensity','Position','Orientation','Color','TextureResourceID'  OutDataTypeStr=Bus: PRESCAN_VISULIGHTACTUATOR_DATA  NonVirtualBus=on
  Bus Creator1 : BusCreator  Inputs=3  OutDataTypeStr=Bus: PRESCAN_RGB_DATA  NonVirtualBus=on
  Bus Creator2 : BusCreator  Inputs=3  OutDataTypeStr=Bus: PRESCAN_RPY_DATA  NonVirtualBus=on
  Bus Creator3 : BusCreator  Inputs=3  OutDataTypeStr=Bus: PRESCAN_XYZ_DATA  NonVirtualBus=on
  Data Type Conversion : DataTypeConversion  OutDataTypeStr=int32  RndMeth=Nearest
  Degrees to Radians : simulink_extras/Transformations/Degrees to Radians
  Demux : Demux  Outputs=3
  Demux1 : Demux  Outputs=3
  Demux2 : Demux  Outputs=3
  Lights : Outport
  wires:
  TextureResourceID [-]/1 -> Data Type Conversion/1  "TextureResourceID"
  MSCD [Cd]/1 -> Bus Creator/1  "Intensity"
  Bus Creator/1 -> Lights/1
  Demux/1 -> Bus Creator1/1  "R"
  Demux/2 -> Bus Creator1/2  "G"
  Demux/3 -> Bus Creator1/3  "B"
  Color [-]/1 -> Demux/1  "Color"
  Bus Creator1/1 -> Bus Creator/4  "Color"
  Demux1/1 -> Bus Creator2/1  "Roll"
  Demux1/2 -> Bus Creator2/2  "Pitch"
  Demux1/3 -> Bus Creator2/3  "Yaw"
  Orientation (RPY) [deg]/1 -> Degrees to Radians/1  "Orientation"
  Bus Creator2/1 -> Bus Creator/3  "Orientation"
  Demux2/1 -> Bus Creator3/1  "X"
  Demux2/2 -> Bus Creator3/2  "Y"
  Demux2/3 -> Bus Creator3/3  "Z"
  Position (xyz) [m]/1 -> Demux2/1  "Position"
  Bus Creator3/1 -> Bus Creator/2  "Position"
  Data Type Conversion/1 -> Bus Creator/5  "TextureResourceID"
  Degrees to Radians/1 -> Demux1/1

== system W01_Base_Map_cs/TrafficLightRoadSideNL_7/Orange_Mux ==
  MSCD [Cd] : Inport
  Position (xyz) [m] : Inport  Port=2
  Orientation (RPY) [deg] : Inport  Port=3
  Color [-] : Inport  Port=4
  TextureResourceID [-] : Inport  Port=5
  Bus Creator : BusCreator  Inputs='Intensity','Position','Orientation','Color','TextureResourceID'  OutDataTypeStr=Bus: PRESCAN_VISULIGHTACTUATOR_DATA  NonVirtualBus=on
  Bus Creator1 : BusCreator  Inputs=3  OutDataTypeStr=Bus: PRESCAN_RGB_DATA  NonVirtualBus=on
  Bus Creator2 : BusCreator  Inputs=3  OutDataTypeStr=Bus: PRESCAN_RPY_DATA  NonVirtualBus=on
  Bus Creator3 : BusCreator  Inputs=3  OutDataTypeStr=Bus: PRESCAN_XYZ_DATA  NonVirtualBus=on
  Data Type Conversion : DataTypeConversion  OutDataTypeStr=int32  RndMeth=Nearest
  Degrees to Radians : simulink_extras/Transformations/Degrees to Radians
  Demux : Demux  Outputs=3
  Demux1 : Demux  Outputs=3
  Demux2 : Demux  Outputs=3
  Lights : Outport
  wires:
  TextureResourceID [-]/1 -> Data Type Conversion/1  "TextureResourceID"
  MSCD [Cd]/1 -> Bus Creator/1  "Intensity"
  Bus Creator/1 -> Lights/1
  Demux/1 -> Bus Creator1/1  "R"
  Demux/2 -> Bus Creator1/2  "G"
  Demux/3 -> Bus Creator1/3  "B"
  Color [-]/1 -> Demux/1  "Color"
  Bus Creator1/1 -> Bus Creator/4  "Color"
  Demux1/1 -> Bus Creator2/1  "Roll"
  Demux1/2 -> Bus Creator2/2  "Pitch"
  Demux1/3 -> Bus Creator2/3  "Yaw"
  Orientation (RPY) [deg]/1 -> Degrees to Radians/1  "Orientation"
  Bus Creator2/1 -> Bus Creator/3  "Orientation"
  Demux2/1 -> Bus Creator3/1  "X"
  Demux2/2 -> Bus Creator3/2  "Y"
  Demux2/3 -> Bus Creator3/3  "Z"
  Position (xyz) [m]/1 -> Demux2/1  "Position"
  Bus Creator3/1 -> Bus Creator/2  "Position"
  Data Type Conversion/1 -> Bus Creator/5  "TextureResourceID"
  Degrees to Radians/1 -> Demux1/1

== system W01_Base_Map_cs/TrafficLightRoadSideNL_7/Red_Mux ==
  MSCD [Cd] : Inport
  Position (xyz) [m] : Inport  Port=2
  Orientation (RPY) [deg] : Inport  Port=3
  Color [-] : Inport  Port=4
  TextureResourceID [-] : Inport  Port=5
  Bus Creator : BusCreator  Inputs='Intensity','Position','Orientation','Color','TextureResourceID'  OutDataTypeStr=Bus: PRESCAN_VISULIGHTACTUATOR_DATA  NonVirtualBus=on
  Bus Creator1 : BusCreator  Inputs=3  OutDataTypeStr=Bus: PRESCAN_RGB_DATA  NonVirtualBus=on
  Bus Creator2 : BusCreator  Inputs=3  OutDataTypeStr=Bus: PRESCAN_RPY_DATA  NonVirtualBus=on
  Bus Creator3 : BusCreator  Inputs=3  OutDataTypeStr=Bus: PRESCAN_XYZ_DATA  NonVirtualBus=on
  Data Type Conversion : DataTypeConversion  OutDataTypeStr=int32  RndMeth=Nearest
  Degrees to Radians : simulink_extras/Transformations/Degrees to Radians
  Demux : Demux  Outputs=3
  Demux1 : Demux  Outputs=3
  Demux2 : Demux  Outputs=3
  Lights : Outport
  wires:
  TextureResourceID [-]/1 -> Data Type Conversion/1  "TextureResourceID"
  MSCD [Cd]/1 -> Bus Creator/1  "Intensity"
  Bus Creator/1 -> Lights/1
  Demux/1 -> Bus Creator1/1  "R"
  Demux/2 -> Bus Creator1/2  "G"
  Demux/3 -> Bus Creator1/3  "B"
  Color [-]/1 -> Demux/1  "Color"
  Bus Creator1/1 -> Bus Creator/4  "Color"
  Demux1/1 -> Bus Creator2/1  "Roll"
  Demux1/2 -> Bus Creator2/2  "Pitch"
  Demux1/3 -> Bus Creator2/3  "Yaw"
  Orientation (RPY) [deg]/1 -> Degrees to Radians/1  "Orientation"
  Bus Creator2/1 -> Bus Creator/3  "Orientation"
  Demux2/1 -> Bus Creator3/1  "X"
  Demux2/2 -> Bus Creator3/2  "Y"
  Demux2/3 -> Bus Creator3/3  "Z"
  Position (xyz) [m]/1 -> Demux2/1  "Position"
  Bus Creator3/1 -> Bus Creator/2  "Position"
  Data Type Conversion/1 -> Bus Creator/5  "TextureResourceID"
  Degrees to Radians/1 -> Demux1/1

== system W01_Base_Map_cs/TrafficLightRoadSideNL_8/Green_Mux ==
  MSCD [Cd] : Inport
  Position (xyz) [m] : Inport  Port=2
  Orientation (RPY) [deg] : Inport  Port=3
  Color [-] : Inport  Port=4
  TextureResourceID [-] : Inport  Port=5
  Bus Creator : BusCreator  Inputs='Intensity','Position','Orientation','Color','TextureResourceID'  OutDataTypeStr=Bus: PRESCAN_VISULIGHTACTUATOR_DATA  NonVirtualBus=on
  Bus Creator1 : BusCreator  Inputs=3  OutDataTypeStr=Bus: PRESCAN_RGB_DATA  NonVirtualBus=on
  Bus Creator2 : BusCreator  Inputs=3  OutDataTypeStr=Bus: PRESCAN_RPY_DATA  NonVirtualBus=on
  Bus Creator3 : BusCreator  Inputs=3  OutDataTypeStr=Bus: PRESCAN_XYZ_DATA  NonVirtualBus=on
  Data Type Conversion : DataTypeConversion  OutDataTypeStr=int32  RndMeth=Nearest
  Degrees to Radians : simulink_extras/Transformations/Degrees to Radians
  Demux : Demux  Outputs=3
  Demux1 : Demux  Outputs=3
  Demux2 : Demux  Outputs=3
  Lights : Outport
  wires:
  TextureResourceID [-]/1 -> Data Type Conversion/1  "TextureResourceID"
  MSCD [Cd]/1 -> Bus Creator/1  "Intensity"
  Bus Creator/1 -> Lights/1
  Demux/1 -> Bus Creator1/1  "R"
  Demux/2 -> Bus Creator1/2  "G"
  Demux/3 -> Bus Creator1/3  "B"
  Color [-]/1 -> Demux/1  "Color"
  Bus Creator1/1 -> Bus Creator/4  "Color"
  Demux1/1 -> Bus Creator2/1  "Roll"
  Demux1/2 -> Bus Creator2/2  "Pitch"
  Demux1/3 -> Bus Creator2/3  "Yaw"
  Orientation (RPY) [deg]/1 -> Degrees to Radians/1  "Orientation"
  Bus Creator2/1 -> Bus Creator/3  "Orientation"
  Demux2/1 -> Bus Creator3/1  "X"
  Demux2/2 -> Bus Creator3/2  "Y"
  Demux2/3 -> Bus Creator3/3  "Z"
  Position (xyz) [m]/1 -> Demux2/1  "Position"
  Bus Creator3/1 -> Bus Creator/2  "Position"
  Data Type Conversion/1 -> Bus Creator/5  "TextureResourceID"
  Degrees to Radians/1 -> Demux1/1

== system W01_Base_Map_cs/TrafficLightRoadSideNL_8/Orange_Mux ==
  MSCD [Cd] : Inport
  Position (xyz) [m] : Inport  Port=2
  Orientation (RPY) [deg] : Inport  Port=3
  Color [-] : Inport  Port=4
  TextureResourceID [-] : Inport  Port=5
  Bus Creator : BusCreator  Inputs='Intensity','Position','Orientation','Color','TextureResourceID'  OutDataTypeStr=Bus: PRESCAN_VISULIGHTACTUATOR_DATA  NonVirtualBus=on
  Bus Creator1 : BusCreator  Inputs=3  OutDataTypeStr=Bus: PRESCAN_RGB_DATA  NonVirtualBus=on
  Bus Creator2 : BusCreator  Inputs=3  OutDataTypeStr=Bus: PRESCAN_RPY_DATA  NonVirtualBus=on
  Bus Creator3 : BusCreator  Inputs=3  OutDataTypeStr=Bus: PRESCAN_XYZ_DATA  NonVirtualBus=on
  Data Type Conversion : DataTypeConversion  OutDataTypeStr=int32  RndMeth=Nearest
  Degrees to Radians : simulink_extras/Transformations/Degrees to Radians
  Demux : Demux  Outputs=3
  Demux1 : Demux  Outputs=3
  Demux2 : Demux  Outputs=3
  Lights : Outport
  wires:
  TextureResourceID [-]/1 -> Data Type Conversion/1  "TextureResourceID"
  MSCD [Cd]/1 -> Bus Creator/1  "Intensity"
  Bus Creator/1 -> Lights/1
  Demux/1 -> Bus Creator1/1  "R"
  Demux/2 -> Bus Creator1/2  "G"
  Demux/3 -> Bus Creator1/3  "B"
  Color [-]/1 -> Demux/1  "Color"
  Bus Creator1/1 -> Bus Creator/4  "Color"
  Demux1/1 -> Bus Creator2/1  "Roll"
  Demux1/2 -> Bus Creator2/2  "Pitch"
  Demux1/3 -> Bus Creator2/3  "Yaw"
  Orientation (RPY) [deg]/1 -> Degrees to Radians/1  "Orientation"
  Bus Creator2/1 -> Bus Creator/3  "Orientation"
  Demux2/1 -> Bus Creator3/1  "X"
  Demux2/2 -> Bus Creator3/2  "Y"
  Demux2/3 -> Bus Creator3/3  "Z"
  Position (xyz) [m]/1 -> Demux2/1  "Position"
  Bus Creator3/1 -> Bus Creator/2  "Position"
  Data Type Conversion/1 -> Bus Creator/5  "TextureResourceID"
  Degrees to Radians/1 -> Demux1/1

== system W01_Base_Map_cs/TrafficLightRoadSideNL_8/Red_Mux ==
  MSCD [Cd] : Inport
  Position (xyz) [m] : Inport  Port=2
  Orientation (RPY) [deg] : Inport  Port=3
  Color [-] : Inport  Port=4
  TextureResourceID [-] : Inport  Port=5
  Bus Creator : BusCreator  Inputs='Intensity','Position','Orientation','Color','TextureResourceID'  OutDataTypeStr=Bus: PRESCAN_VISULIGHTACTUATOR_DATA  NonVirtualBus=on
  Bus Creator1 : BusCreator  Inputs=3  OutDataTypeStr=Bus: PRESCAN_RGB_DATA  NonVirtualBus=on
  Bus Creator2 : BusCreator  Inputs=3  OutDataTypeStr=Bus: PRESCAN_RPY_DATA  NonVirtualBus=on
  Bus Creator3 : BusCreator  Inputs=3  OutDataTypeStr=Bus: PRESCAN_XYZ_DATA  NonVirtualBus=on
  Data Type Conversion : DataTypeConversion  OutDataTypeStr=int32  RndMeth=Nearest
  Degrees to Radians : simulink_extras/Transformations/Degrees to Radians
  Demux : Demux  Outputs=3
  Demux1 : Demux  Outputs=3
  Demux2 : Demux  Outputs=3
  Lights : Outport
  wires:
  TextureResourceID [-]/1 -> Data Type Conversion/1  "TextureResourceID"
  MSCD [Cd]/1 -> Bus Creator/1  "Intensity"
  Bus Creator/1 -> Lights/1
  Demux/1 -> Bus Creator1/1  "R"
  Demux/2 -> Bus Creator1/2  "G"
  Demux/3 -> Bus Creator1/3  "B"
  Color [-]/1 -> Demux/1  "Color"
  Bus Creator1/1 -> Bus Creator/4  "Color"
  Demux1/1 -> Bus Creator2/1  "Roll"
  Demux1/2 -> Bus Creator2/2  "Pitch"
  Demux1/3 -> Bus Creator2/3  "Yaw"
  Orientation (RPY) [deg]/1 -> Degrees to Radians/1  "Orientation"
  Bus Creator2/1 -> Bus Creator/3  "Orientation"
  Demux2/1 -> Bus Creator3/1  "X"
  Demux2/2 -> Bus Creator3/2  "Y"
  Demux2/3 -> Bus Creator3/3  "Z"
  Position (xyz) [m]/1 -> Demux2/1  "Position"
  Bus Creator3/1 -> Bus Creator/2  "Position"
  Data Type Conversion/1 -> Bus Creator/5  "TextureResourceID"
  Degrees to Radians/1 -> Demux1/1

== system W01_Base_Map_cs/Audi_A8_Sedan_1/SELF_Demux/compas converter ==
  rotz [rad] : Inport
  cart2compas : Subsystem
  rad2deg : Gain  Gain=180/pi
  heading [deg] : Outport
  wires:
  rad2deg/1 -> cart2compas/1(Angle [deg])
  rotz [rad]/1 -> rad2deg/1
  cart2compas/1(heading [deg]) -> heading [deg]/1

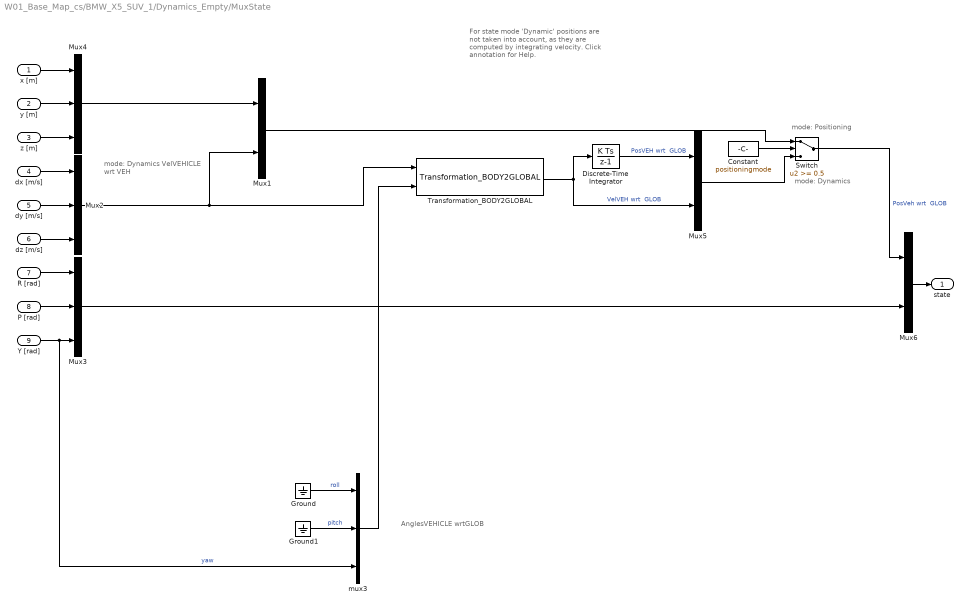
== system W01_Base_Map_cs/BMW_X5_SUV_1/Dynamics_Empty/MuxState ==
  note: mode: Dynamics
  note: mode: Positioning
  note: mode: Dynamics
      | VelVEHICLE
      | wrt VEH
  note: AnglesVEHICLE
      | wrtGLOB
  note: For state mode 'Dynamic' positions
      | are not taken into account, as they
      | are computed by integrating velocity.
      | Click annotation for Help.
  x [m] : Inport  SampleTime=TimeStep
  y [m] : Inport  Port=2  SampleTime=TimeStep
  z [m] : Inport  Port=3  SampleTime=TimeStep
  dx [m/s] : Inport  Port=4  SampleTime=TimeStep
  dy [m/s] : Inport  Port=5  SampleTime=TimeStep
  dz [m/s] : Inport  Port=6  SampleTime=TimeStep
  R [rad] : Inport  Port=7  SampleTime=TimeStep
  P [rad] : Inport  Port=8  SampleTime=TimeStep
  Y [rad] : Inport  Port=9  SampleTime=TimeStep
  Constant : Constant  DisableCoverage=on  Value=positioningmode
  Discrete-Time Integrator : DiscreteIntegrator  SampleTime=TimeStep  ICPrevOutput=DiscIntNeverNeededParam  ICPrevScaledInput=DiscIntNeverNeededParam
  Ground : Ground
  Ground1 : Ground
  Mux1 : Mux  Inputs=[3 3]
  Mux2 : Mux  Inputs=3
  Mux3 : Mux  Inputs=3
  Mux4 : Mux  Inputs=3
  Mux5 : Mux  Inputs=[3 3]
  Mux6 : Mux  Inputs=[6 3]
  Switch : Switch  Threshold=0.5
  Transformation_BODY2GLOBAL : PreScanSimulinkLibrary/Simple_Vehicle_Dynamics/Chassis/MuxDynState/Transformation_BODY2GLOBAL  SystemSampleTime=-1
  mux3 : Mux  Inputs=3
  state : Outport
  wires:
  Constant/1 -> Switch/2
  Mux6/1 -> state/1
  Mux4/1 -> Mux1/1
  Mux5/1 -> Switch/3
  Mux1/1 -> Switch/1
  Switch/1 -> Mux6/1  "PosVeh wrt  GLOB"
  P [rad]/1 -> Mux3/2
  R [rad]/1 -> Mux3/1
  dz [m/s]/1 -> Mux2/3
  dy [m/s]/1 -> Mux2/2
  dx [m/s]/1 -> Mux2/1
  z [m]/1 -> Mux4/3
  y [m]/1 -> Mux4/2
  x [m]/1 -> Mux4/1
  Ground1/1 -> mux3/2  "pitch"
  Y [rad]/1 -> mux3/3, Mux3/3  "yaw"
  Mux3/1 -> Mux6/2
  Transformation_BODY2GLOBAL/1 -> Discrete-Time Integrator/1, Mux5/2  "VelVEH wrt  GLOB"
  mux3/1 -> Transformation_BODY2GLOBAL/2
  Ground/1 -> mux3/1  "roll"
  Mux2/1 -> Mux1/2, Transformation_BODY2GLOBAL/1
  Discrete-Time Integrator/1 -> Mux5/1  "PosVEH wrt  GLOB"

== system W01_Base_Map_cs/BMW_X5_SUV_1/Dynamics_Empty/STATE_BMW_X5_SUV_1 ==
  State : Inport  SampleTime=TimeStep
  Bus Creator : BusCreator  Inputs=15  OutDataTypeStr=Bus: PRESCAN_STATEACTUATORDATA  NonVirtualBus=on
  Constant : Constant  Value=0
  Demux : Demux  Outputs=15
  Mux : Mux  Inputs=3
  Mux1 : Mux  Inputs=3
  Mux2 : Mux  Inputs=3
  iniBODYAngles wrtVEH [rad] : Constant  Value=Roll0  SampleTime=TimeStep
  iniBODYAngles wrtVEH [rad]1 : Constant  Value=Pitch0  SampleTime=TimeStep
  iniVEHAngles wrtGLOB [rad] : Constant  Value=Yaw0  SampleTime=TimeStep
  iniVEHposition wrtGLOB [m] : Constant  Value=x0  SampleTime=TimeStep
  iniVEHposition wrtGLOB [m]1 : Constant  Value=y0  SampleTime=TimeStep
  iniVEHposition wrtGLOB [m]2 : Constant  Value=z0  SampleTime=TimeStep
  state2FullState : PreScanSimulinkLibrary/state2FullState  SystemSampleTime=-1
  StateBus : Outport  OutDataTypeStr=Bus: PRESCAN_STATEACTUATORDATA
  wires:
  Mux2/1 -> state2FullState/4
  iniVEHAngles wrtGLOB [rad]/1 -> Mux2/3
  Mux1/1 -> state2FullState/3
  Constant/1 -> Mux2/1, Mux2/2, Mux1/3
  iniBODYAngles wrtVEH [rad]1/1 -> Mux1/2
  iniBODYAngles wrtVEH [rad]/1 -> Mux1/1
  Mux/1 -> state2FullState/2
  iniVEHposition wrtGLOB [m]2/1 -> Mux/3
  iniVEHposition wrtGLOB [m]/1 -> Mux/1
  iniVEHposition wrtGLOB [m]1/1 -> Mux/2
  Demux/15 -> Bus Creator/15  "AngularVelocityYaw"
  Demux/14 -> Bus Creator/14  "AngularVelocityPitch"
  Demux/13 -> Bus Creator/13  "AngularVelocityRoll"
  Demux/12 -> Bus Creator/12  "OrientationYaw"
  Demux/11 -> Bus Creator/11  "OrientationPitch"
  Demux/10 -> Bus Creator/10  "OrientationRoll"
  Demux/9 -> Bus Creator/9  "AccelerationZ"
  Demux/8 -> Bus Creator/8  "AccelerationY"
  Demux/7 -> Bus Creator/7  "AccelerationX"
  Demux/6 -> Bus Creator/6  "VelocityZ"
  Demux/5 -> Bus Creator/5  "VelocityY"
  Demux/4 -> Bus Creator/4  "VelocityX"
  Demux/3 -> Bus Creator/3  "PositionZ"
  Demux/2 -> Bus Creator/2  "PositionY"
  Demux/1 -> Bus Creator/1  "PositionX"
  state2FullState/1 -> Demux/1
  State/1 -> state2FullState/1
  Bus Creator/1 -> StateBus/1

== system W01_Base_Map_cs/BMW_X5_SUV_1/SELF_Demux/compas converter ==
  rotz [rad] : Inport
  cart2compas : Subsystem
  rad2deg : Gain  Gain=180/pi
  heading [deg] : Outport
  wires:
  rad2deg/1 -> cart2compas/1(Angle [deg])
  rotz [rad]/1 -> rad2deg/1
  cart2compas/1(heading [deg]) -> heading [deg]/1

== system W01_Base_Map_cs/Child_RegularAni_1/Animation/animation mode ==
  vel : Inport
  Data Type Conversion : DataTypeConversion  OutDataTypeStr=double
  Fcn : Fcn  Expr=sqrt(u(1)^2+u(2)^2+u(3)^2)
  Running : simulink/Logic and Bit Operations/Compare To Constant  relop=>=  const=MWS  OutDataTypeStr=uint8  ZeroCross=off
  Sum : Sum  Inputs=|++
  Walking : simulink/Logic and Bit Operations/Compare To Zero  relop=~=  OutDataTypeStr=uint8  ZeroCross=off
  mode : Outport
  wires:
  vel/1 -> Fcn/1
  Sum/1 -> Data Type Conversion/1
  Walking/1 -> Sum/1
  Running/1 -> Sum/2
  Fcn/1 -> Walking/1, Running/1
  Data Type Conversion/1 -> mode/1

== system W01_Base_Map_cs/Child_RegularAni_1/Animation/elapsed track ==
  vel : Inport
  Discrete-Time Integrator : DiscreteIntegrator  SampleTime=-1  ICPrevOutput=DiscIntNeverNeededParam  ICPrevScaledInput=DiscIntNeverNeededParam
  Fcn : Fcn  Expr=sqrt(u(1)^2 + u(2)^2 + u(3)^2)
  s : Outport
  wires:
  Fcn/1 -> Discrete-Time Integrator/1
  vel/1 -> Fcn/1
  Discrete-Time Integrator/1 -> s/1

== system W01_Base_Map_cs/Child_RegularAni_1/SELF_Demux/compas converter ==
  rotz [rad] : Inport
  cart2compas : Subsystem
  rad2deg : Gain  Gain=180/pi
  heading [deg] : Outport
  wires:
  rad2deg/1 -> cart2compas/1(Angle [deg])
  rotz [rad]/1 -> rad2deg/1
  cart2compas/1(heading [deg]) -> heading [deg]/1

== system W01_Base_Map_cs/Child_RegularAni_2/Animation/animation mode ==
  vel : Inport
  Data Type Conversion : DataTypeConversion  OutDataTypeStr=double
  Fcn : Fcn  Expr=sqrt(u(1)^2+u(2)^2+u(3)^2)
  Running : simulink/Logic and Bit Operations/Compare To Constant  relop=>=  const=MWS  OutDataTypeStr=uint8  ZeroCross=off
  Sum : Sum  Inputs=|++
  Walking : simulink/Logic and Bit Operations/Compare To Zero  relop=~=  OutDataTypeStr=uint8  ZeroCross=off
  mode : Outport
  wires:
  vel/1 -> Fcn/1
  Sum/1 -> Data Type Conversion/1
  Walking/1 -> Sum/1
  Running/1 -> Sum/2
  Fcn/1 -> Walking/1, Running/1
  Data Type Conversion/1 -> mode/1
